simulink model "controller"  (R2022b)
settings: Solver=VariableStepAuto  StartTime=0.0  StopTime=10  RelTol=1e-3
values from neighbouring files (symbols this model uses):
  a_1 = x(25)    [disturbance_torque_generator.m]    (also in dynamic_terms.m = robot_parameters(9); dz_calculator.m; load_data.m = 0.5; nonlinear_disturbance_observer_controller.m)
  a_2 = x(26)    [disturbance_torque_generator.m]    (also in dynamic_terms.m = robot_parameters(10); dz_calculator.m; load_data.m = 0.4; nonlinear_disturbance_observer_controller.m)
  f_c1 = x(5)    [disturbance_torque_generator.m]    (also in load_data.m = 0.49)
  f_c2 = x(6)    [disturbance_torque_generator.m]    (also in load_data.m = 0.31)
  f_c3 = x(7)    [disturbance_torque_generator.m]    (also in load_data.m = 0.1)
  f_c4 = x(8)    [disturbance_torque_generator.m]    (also in load_data.m = 0.1)
  f_payload = x(27)    [disturbance_torque_generator.m]    (also in load_data.m = 2)
  f_s1 = x(9)    [disturbance_torque_generator.m]    (also in load_data.m = 3.5)
  f_s2 = x(10)    [disturbance_torque_generator.m]    (also in load_data.m = 2.8)
  f_s3 = x(11)    [disturbance_torque_generator.m]    (also in load_data.m = 1.65)
  f_s4 = x(12)    [disturbance_torque_generator.m]    (also in load_data.m = 0.7)
  f_v1 = x(13)    [disturbance_torque_generator.m]    (also in load_data.m = 0.15)
  f_v2 = x(14)    [disturbance_torque_generator.m]    (also in load_data.m = 0.12)
  f_v3 = x(15)    [disturbance_torque_generator.m]    (also in load_data.m = 0.08)
  f_v4 = x(16)    [disturbance_torque_generator.m]    (also in load_data.m = 0.03)
  I_1 = robot_parameters(5)    [dynamic_terms.m]    (also in dz_calculator.m = x(21); load_data.m = 0.31305; nonlinear_disturbance_observer_controller.m = x(21); open_loop_dynamics.m = x(17))
  I_2 = robot_parameters(6)    [dynamic_terms.m]    (also in dz_calculator.m = x(22); load_data.m = 0.96; nonlinear_disturbance_observer_controller.m = x(22); open_loop_dynamics.m = x(18))
  I_3 = robot_parameters(7)    [dynamic_terms.m]    (also in dz_calculator.m = x(23); load_data.m = 0.05; nonlinear_disturbance_observer_controller.m = x(23); open_loop_dynamics.m = x(19))
  I_4 = robot_parameters(8)    [dynamic_terms.m]    (also in dz_calculator.m = x(24); load_data.m = 0.06; nonlinear_disturbance_observer_controller.m = x(24); open_loop_dynamics.m = x(20))
  k_p = 2    [load_data.m]    (also in nonlinear_disturbance_observer_controller.m = x(30))
  k_v = 1.5    [load_data.m]    (also in nonlinear_disturbance_observer_controller.m = x(29))
  m_1 = robot_parameters(1)    [dynamic_terms.m]    (also in dz_calculator.m = x(17); load_data.m = 15; nonlinear_disturbance_observer_controller.m = x(17); open_loop_dynamics.m = x(13))
  m_2 = robot_parameters(2)    [dynamic_terms.m]    (also in dz_calculator.m = x(18); load_data.m = 12; nonlinear_disturbance_observer_controller.m = x(18); open_loop_dynamics.m = x(14))
  m_3 = robot_parameters(3)    [dynamic_terms.m]    (also in dz_calculator.m = x(19); load_data.m = 3; nonlinear_disturbance_observer_controller.m = x(19); open_loop_dynamics.m = x(15))
  m_4 = robot_parameters(4)    [dynamic_terms.m]    (also in dz_calculator.m = x(20); load_data.m = 3; nonlinear_disturbance_observer_controller.m = x(20); open_loop_dynamics.m = x(16))
  v_s1 = x(17)    [disturbance_torque_generator.m]    (also in load_data.m = 0.19)
  v_s2 = x(18)    [disturbance_torque_generator.m]    (also in load_data.m = 0.15)
  v_s3 = x(19)    [disturbance_torque_generator.m]    (also in load_data.m = 0.12)
  v_s4 = x(20)    [disturbance_torque_generator.m]    (also in load_data.m = 0.03)
  x_1 = robot_parameters(11)    [dynamic_terms.m]    (also in dz_calculator.m = x(27); load_data.m = 0.25; nonlinear_disturbance_observer_controller.m = x(27); open_loop_dynamics.m = x(23))
  x_2 = robot_parameters(12)    [dynamic_terms.m]    (also in dz_calculator.m = x(28); load_data.m = 0.2; nonlinear_disturbance_observer_controller.m = x(28); open_loop_dynamics.m = x(24))
  x_inv = x(5)    [dp_calculator.m]    (also in dz_calculator.m = x(29); load_data.m = 95.8)
libraries: simulink x8
settings Model: Creator=Mahdi  LastModifiedBy=Mahdi
settings SolverCC: MaxConsecutiveMinStep=10
settings DebuggingCC: UnderSpecifiedDimensionMsg=warning

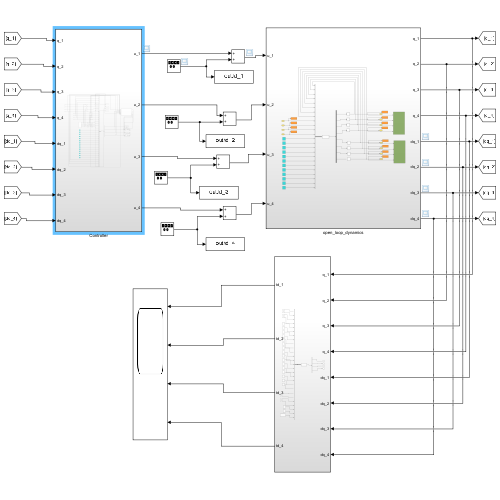
[thumbnail: Simulink's stored preview of the top-level diagram]
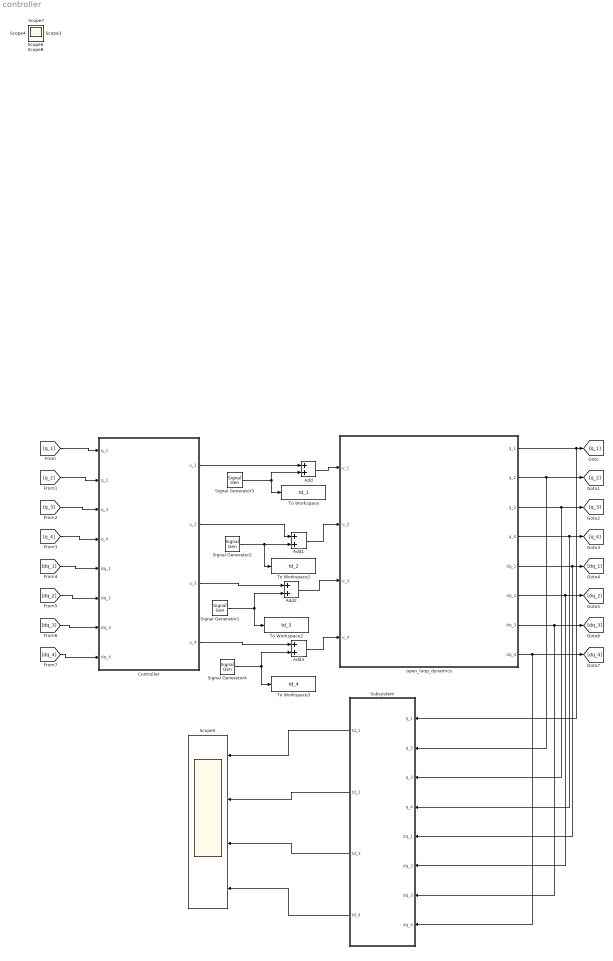
== system controller ==
  Add{,1..3} (4 alike) : Sum
  Controller : Subsystem
  Scope5 : Scope  NumInputPorts=4
  Signal Generator1 : SignalGenerator  Amplitude=0  Frequency=18  Units=rad/sec
  Signal Generator2 : SignalGenerator  Amplitude=-0.4  Frequency=0.8  Units=rad/sec
  Signal Generator3 : SignalGenerator  Amplitude=0.2  Frequency=0.27  Units=rad/sec
  Signal Generator4 : SignalGenerator  Amplitude=0  Frequency=4  Units=rad/sec
  Subsystem : Subsystem
  To Workspace : ToWorkspace  VariableName=td_1  SaveFormat=Timeseries  SampleTime=-1
  To Workspace1 : ToWorkspace  VariableName=td_2  SaveFormat=Timeseries  SampleTime=-1
  To Workspace2 : ToWorkspace  VariableName=td_3  SaveFormat=Timeseries  SampleTime=-1
  To Workspace3 : ToWorkspace  VariableName=td_4  SaveFormat=Timeseries  SampleTime=-1
  open_loop_dynamics : Subsystem
  Scope{,1..4,6..8} (8 alike) : Scope
  wires:
  [q_1] -> Controller/1(q_1)
  [q_2] -> Controller/2(q_2)
  [q_3] -> Controller/3(q_3)
  [q_4] -> Controller/4(q_4)
  [dq_1] -> Controller/5(dq_1)
  [dq_2] -> Controller/6(dq_2)
  [dq_3] -> Controller/7(dq_3)
  [dq_4] -> Controller/8(dq_4)
  open_loop_dynamics/1(q_1) -> Subsystem/1(q_1), [q_1]
  open_loop_dynamics/2(q_2) -> [q_2], Subsystem/2(q_2)
  open_loop_dynamics/3(q_3) -> [q_3], Subsystem/3(q_3)
  open_loop_dynamics/4(q_4) -> [q_4], Subsystem/4(q_4)
  open_loop_dynamics/5(dq_1) -> [dq_1], Subsystem/5(dq_1)
  open_loop_dynamics/6(dq_2) -> [dq_2], Subsystem/6(dq_2)
  open_loop_dynamics/7(dq_3) -> [dq_3], Subsystem/7(dq_3)
  open_loop_dynamics/8(dq_4) -> [dq_4], Subsystem/8(dq_4)
  Signal Generator3/1 -> Add/2, To Workspace/1
  Signal Generator2/1 -> Add1/2, To Workspace1/1
  Signal Generator1/1 -> Add2/2, To Workspace2/1
  Controller/1(u_1) -> Add/1
  Controller/2(u_2) -> Add1/1
  Add/1 -> open_loop_dynamics/1(u_1)
  Add1/1 -> open_loop_dynamics/2(u_2)
  Add2/1 -> open_loop_dynamics/3(u_3)
  Controller/3(u_3) -> Add2/1
  Signal Generator4/1 -> Add3/2, To Workspace3/1
  Controller/4(u_4) -> Add3/1
  Add3/1 -> open_loop_dynamics/4(u_4)
  Subsystem/1(td_1) -> Scope5/1
  Subsystem/2(td_2) -> Scope5/2
  Subsystem/3(td_3) -> Scope5/3
  Subsystem/4(td_4) -> Scope5/4

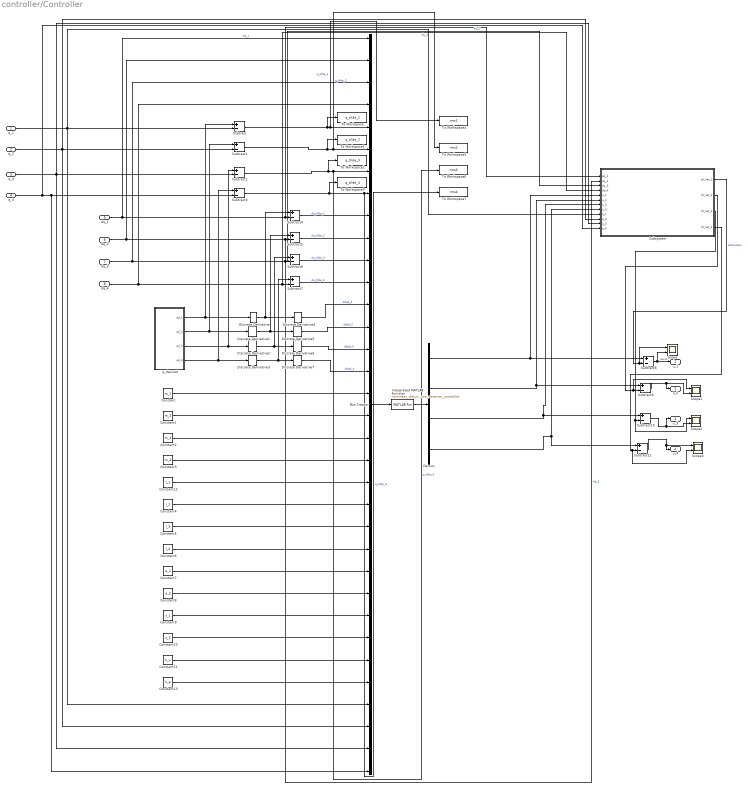
== system controller/Controller ==
  q_1 : Inport
  q_2 : Inport  Port=2
  q_3 : Inport  Port=3
  q_4 : Inport  Port=4
  dq_1 : Inport  Port=5
  dq_2 : Inport  Port=6
  dq_3 : Inport  Port=7
  dq_4 : Inport  Port=8
  Bus Creator : BusCreator  Inputs=34
  Constant : Constant  Value=m_1
  Constant1 : Constant  Value=m_2
  Constant10 : Constant  Value=x_2
  Constant11 : Constant  Value=k_v
  Constant12 : Constant  Value=I_1
  Constant13 : Constant  Value=k_p
  Constant2 : Constant  Value=m_3
  Constant3 : Constant  Value=m_4
  Constant4 : Constant  Value=I_2
  Constant5 : Constant  Value=I_3
  Constant6 : Constant  Value=I_4
  Constant7 : Constant  Value=a_1
  Constant8 : Constant  Value=a_2
  Constant9 : Constant  Value=x_1
  Demux : Demux
  Discrete Derivative{,1..7} (8 alike) : simulink/Discrete/Discrete Derivative  gainval=1.0  ICPrevScaledInput=0.0  OutMin=[]  OutMax=[]  OutDataType=fixdt(1, 16)  OutScaling=2^-10  DoSatur=off
  Interpreted MATLAB Function : MATLABFcn  MATLABFcn=nonlinear_disturbance_observer_controller
  Scope{,1..3} (4 alike) : Scope  NumInputPorts=2
  Subsystem : Subsystem
  Subtract{,1..11} (12 alike) : Sum  Inputs=+-
  To Workspace : ToWorkspace  VariableName=q_tilde_1  SaveFormat=Timeseries  SampleTime=-1
  To Workspace1 : ToWorkspace  VariableName=q_tilde_2  SaveFormat=Timeseries  SampleTime=-1
  To Workspace2 : ToWorkspace  VariableName=q_tilde_3  SaveFormat=Timeseries  SampleTime=-1
  To Workspace3 : ToWorkspace  VariableName=q_tilde_4  SaveFormat=Timeseries  SampleTime=-1
  To Workspace4 : ToWorkspace  VariableName=rms1  SampleTime=-1
      settings: Save2DSignal=2-D array (concatenate along first dimension)
  To Workspace5 : ToWorkspace  VariableName=rms2  SampleTime=-1
      settings: Save2DSignal=2-D array (concatenate along first dimension)
  To Workspace6 : ToWorkspace  VariableName=rms3  SampleTime=-1
      settings: Save2DSignal=2-D array (concatenate along first dimension)
  To Workspace7 : ToWorkspace  VariableName=rms4  SampleTime=-1
      settings: Save2DSignal=2-D array (concatenate along first dimension)
  q_desired : Subsystem
  u_1 : Outport
  u_2 : Outport  Port=2
  u_3 : Outport  Port=3
  u_4 : Outport  Port=4
  wires:
  dq_2/1 -> Bus Creator/2, Subsystem/2(dq_2), Subtract5/2  "dq_2"
  dq_1/1 -> Bus Creator/1, Subsystem/1(dq_1), Subtract4/2  "dq_1"
  q_desired/1(qd_1) -> Discrete Derivative/1, Subtract/1
  q_desired/4(qd_4) -> Discrete Derivative3/1, Subtract3/1
  dq_3/1 -> Bus Creator/3, Subsystem/3(dq_3), Subtract6/2  "dq_3"
  Discrete Derivative5/1 -> Bus Creator/14  "ddqd_2"
  Discrete Derivative/1 -> Discrete Derivative4/1, Subtract4/1
  Discrete Derivative3/1 -> Discrete Derivative7/1, Subtract7/1
  Subtract3/1 -> To Workspace7/1, Bus Creator/8, To Workspace3/1  "q_tilde_4"
  Interpreted MATLAB Function/1 -> Demux/1
  Constant3/1 -> Bus Creator/20
  q_desired/2(qd_2) -> Discrete Derivative1/1, Subtract1/1
  q_1/1 -> Subtract/2, Bus Creator/31, Subsystem/9(q_1)
  Constant/1 -> Bus Creator/17
  Constant12/1 -> Bus Creator/21
  Constant6/1 -> Bus Creator/24
  Constant2/1 -> Bus Creator/19
  Subtract4/1 -> Bus Creator/9  "dq_tilde_1"
  Constant9/1 -> Bus Creator/27
  Subtract6/1 -> Bus Creator/11  "dq_tilde_3"
  Discrete Derivative6/1 -> Bus Creator/15  "ddqd_3"
  Constant5/1 -> Bus Creator/23
  dq_4/1 -> Bus Creator/4, Subtract7/2, Subsystem/4(dq_4)  "dq_4"
  Constant11/1 -> Bus Creator/29
  Constant4/1 -> Bus Creator/22
  Discrete Derivative7/1 -> Bus Creator/16  "ddqd_4"
  Discrete Derivative4/1 -> Bus Creator/13  "ddqd_1"
  Constant8/1 -> Bus Creator/26
  Subtract5/1 -> Bus Creator/10  "dq_tilde_2"
  Discrete Derivative1/1 -> Discrete Derivative5/1, Subtract5/1
  q_3/1 -> Subtract2/2, Bus Creator/33, Subsystem/11(q_3)
  Subtract1/1 -> To Workspace1/1, Bus Creator/6, To Workspace5/1  "q_tilde_2"
  Subtract7/1 -> Bus Creator/12  "dq_tilde_4"
  Subtract/1 -> To Workspace4/1, Bus Creator/5, To Workspace/1  "q_tilde_1"
  q_4/1 -> Subsystem/12(q_4), Bus Creator/34, Subtract3/2
  q_desired/3(qd_3) -> Discrete Derivative2/1, Subtract2/1
  Discrete Derivative2/1 -> Discrete Derivative6/1, Subtract6/1
  Constant10/1 -> Bus Creator/28
  q_2/1 -> Subtract1/2, Bus Creator/32, Subsystem/10(q_2)
  Subtract2/1 -> To Workspace6/1, Bus Creator/7, To Workspace2/1  "q_tilde_3"
  Constant1/1 -> Bus Creator/18
  Constant7/1 -> Bus Creator/25
  Constant13/1 -> Bus Creator/30
  Bus Creator/1 -> Interpreted MATLAB Function/1
  Demux/1 -> Subtract8/1, Subsystem/5(u_1)
  Subsystem/1(td_hat_1) -> Scope/1, Subtract8/2  "estimation"
  Demux/2 -> Subtract9/1, Subsystem/6(u_2)
  Demux/3 -> Subtract10/1, Subsystem/7(u_3)
  Demux/4 -> Subtract11/1, Subsystem/8(u_4)
  Subsystem/2(td_hat_2) -> Subtract9/2, Scope1/1
  Subsystem/3(td_hat_3) -> Scope2/1, Subtract10/2
  Subsystem/4(td_hat_4) -> Scope3/2, Subtract11/2
  Subtract8/1 -> u_1/1, Scope/2  "result"
  Subtract10/1 -> u_3/1, Scope2/2
  Subtract9/1 -> u_2/1, Scope1/2
  Subtract11/1 -> u_4/1, Scope3/1

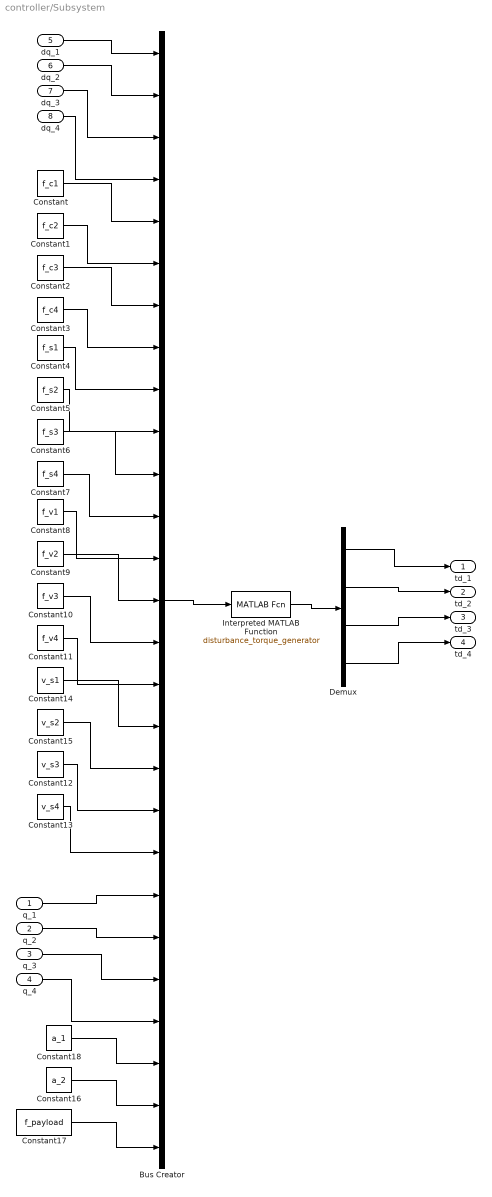
== system controller/Subsystem ==
  q_1 : Inport
  q_2 : Inport  Port=2
  q_3 : Inport  Port=3
  q_4 : Inport  Port=4
  dq_1 : Inport  Port=5
  dq_2 : Inport  Port=6
  dq_3 : Inport  Port=7
  dq_4 : Inport  Port=8
  Bus Creator : BusCreator  Inputs=27
  Constant : Constant  Value=f_c1
  Constant1 : Constant  Value=f_c2
  Constant10 : Constant  Value=f_v3
  Constant11 : Constant  Value=f_v4
  Constant12 : Constant  Value=v_s3
  Constant13 : Constant  Value=v_s4
  Constant14 : Constant  Value=v_s1
  Constant15 : Constant  Value=v_s2
  Constant16 : Constant  Value=a_2
  Constant17 : Constant  Value=f_payload
  Constant18 : Constant  Value=a_1
  Constant2 : Constant  Value=f_c3
  Constant3 : Constant  Value=f_c4
  Constant4 : Constant  Value=f_s1
  Constant5 : Constant  Value=f_s2
  Constant6 : Constant  Value=f_s3
  Constant7 : Constant  Value=f_s4
  Constant8 : Constant  Value=f_v1
  Constant9 : Constant  Value=f_v2
  Demux : Demux
  Interpreted MATLAB Function : MATLABFcn  MATLABFcn=disturbance_torque_generator
  td_1 : Outport
  td_2 : Outport  Port=2
  td_3 : Outport  Port=3
  td_4 : Outport  Port=4
  wires:
  Constant/1 -> Bus Creator/5
  Constant1/1 -> Bus Creator/6
  Constant2/1 -> Bus Creator/7
  Constant3/1 -> Bus Creator/8
  Constant4/1 -> Bus Creator/9
  Constant5/1 -> Bus Creator/10
  Constant6/1 -> Bus Creator/11
  Constant7/1 -> Bus Creator/12
  Constant8/1 -> Bus Creator/13
  Constant9/1 -> Bus Creator/14
  Constant10/1 -> Bus Creator/15
  Constant11/1 -> Bus Creator/16
  Constant14/1 -> Bus Creator/17
  Constant15/1 -> Bus Creator/18
  Constant12/1 -> Bus Creator/19
  Constant13/1 -> Bus Creator/20
  Constant17/1 -> Bus Creator/27
  Constant16/1 -> Bus Creator/26
  Constant18/1 -> Bus Creator/25
  dq_1/1 -> Bus Creator/1
  dq_2/1 -> Bus Creator/2
  dq_3/1 -> Bus Creator/3
  dq_4/1 -> Bus Creator/4
  q_1/1 -> Bus Creator/21
  q_2/1 -> Bus Creator/22
  q_3/1 -> Bus Creator/23
  q_4/1 -> Bus Creator/24
  Bus Creator/1 -> Interpreted MATLAB Function/1
  Interpreted MATLAB Function/1 -> Demux/1
  Demux/1 -> td_1/1
  Demux/2 -> td_2/1
  Demux/3 -> td_3/1
  Demux/4 -> td_4/1

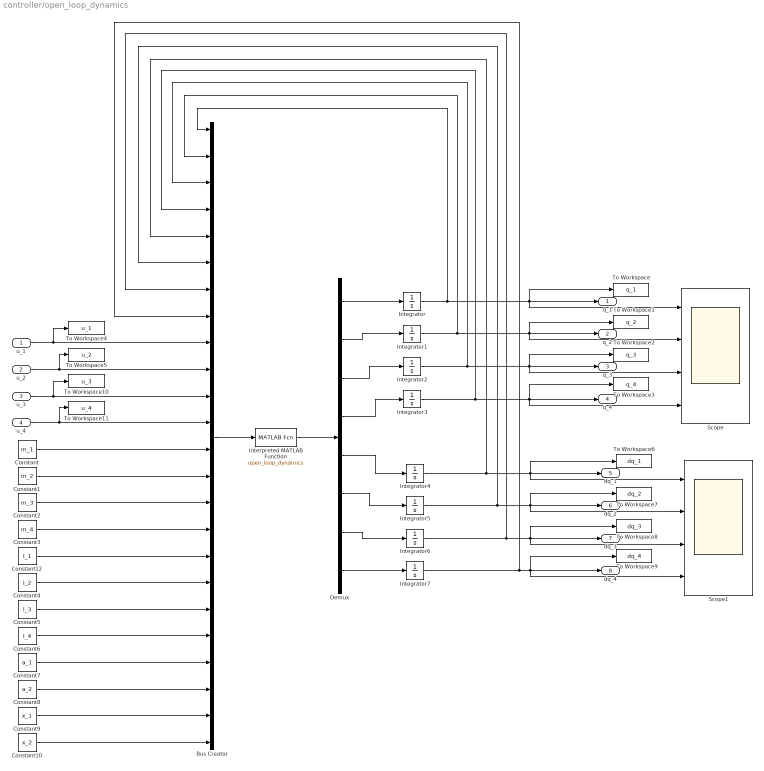
== system controller/open_loop_dynamics ==
  u_1 : Inport
  u_2 : Inport  Port=2
  u_3 : Inport  Port=3
  u_4 : Inport  Port=4
  Bus Creator : BusCreator  Inputs=24
  Constant : Constant  Value=m_1
  Constant1 : Constant  Value=m_2
  Constant10 : Constant  Value=x_2
  Constant12 : Constant  Value=I_1
  Constant2 : Constant  Value=m_3
  Constant3 : Constant  Value=m_4
  Constant4 : Constant  Value=I_2
  Constant5 : Constant  Value=I_3
  Constant6 : Constant  Value=I_4
  Constant7 : Constant  Value=a_1
  Constant8 : Constant  Value=a_2
  Constant9 : Constant  Value=x_1
  Demux : Demux  Outputs=8
  Integrator{,1..7} (8 alike) : Integrator
  Interpreted MATLAB Function : MATLABFcn  MATLABFcn=open_loop_dynamics
  Scope : Scope  NumInputPorts=4
  Scope1 : Scope  NumInputPorts=4
  To Workspace : ToWorkspace  VariableName=q_1  SampleTime=-1
  To Workspace1 : ToWorkspace  VariableName=q_2  SampleTime=-1
  To Workspace10 : ToWorkspace  VariableName=u_3  SampleTime=-1
  To Workspace11 : ToWorkspace  VariableName=u_4  SampleTime=-1
  To Workspace2 : ToWorkspace  VariableName=q_3  SampleTime=-1
  To Workspace3 : ToWorkspace  VariableName=q_4  SampleTime=-1
  To Workspace4 : ToWorkspace  VariableName=u_1  SampleTime=-1
  To Workspace5 : ToWorkspace  VariableName=u_2  SampleTime=-1
  To Workspace6 : ToWorkspace  VariableName=dq_1  SampleTime=-1
  To Workspace7 : ToWorkspace  VariableName=dq_2  SampleTime=-1
  To Workspace8 : ToWorkspace  VariableName=dq_3  SampleTime=-1
  To Workspace9 : ToWorkspace  VariableName=dq_4  SampleTime=-1
  q_1 : Outport
  q_2 : Outport  Port=2
  q_3 : Outport  Port=3
  q_4 : Outport  Port=4
  dq_1 : Outport  Port=5
  dq_2 : Outport  Port=6
  dq_3 : Outport  Port=7
  dq_4 : Outport  Port=8
  wires:
  Integrator6/1 -> dq_3/1, Scope1/3, To Workspace8/1, Bus Creator/7
  Integrator/1 -> q_1/1, To Workspace/1, Scope/1, Bus Creator/1
  Constant3/1 -> Bus Creator/16
  Integrator4/1 -> dq_1/1, Scope1/1, To Workspace6/1, Bus Creator/5
  Constant5/1 -> Bus Creator/19
  u_2/1 -> To Workspace5/1, Bus Creator/10
  Demux/3 -> Integrator2/1
  u_4/1 -> Bus Creator/12, To Workspace11/1
  Constant4/1 -> Bus Creator/18
  u_1/1 -> Bus Creator/9, To Workspace4/1
  Demux/4 -> Integrator3/1
  Integrator2/1 -> q_3/1, To Workspace2/1, Scope/3, Bus Creator/3
  Integrator3/1 -> q_4/1, To Workspace3/1, Scope/4, Bus Creator/4
  Integrator7/1 -> dq_4/1, Scope1/4, To Workspace9/1, Bus Creator/8
  Demux/1 -> Integrator/1
  Constant2/1 -> Bus Creator/15
  Demux/7 -> Integrator6/1
  Interpreted MATLAB Function/1 -> Demux/1
  Demux/2 -> Integrator1/1
  Integrator5/1 -> dq_2/1, Scope1/2, To Workspace7/1, Bus Creator/6
  Demux/8 -> Integrator7/1
  Demux/6 -> Integrator5/1
  Integrator1/1 -> q_2/1, To Workspace1/1, Scope/2, Bus Creator/2
  u_3/1 -> Bus Creator/11, To Workspace10/1
  Bus Creator/1 -> Interpreted MATLAB Function/1
  Demux/5 -> Integrator4/1
  Constant12/1 -> Bus Creator/17
  Constant6/1 -> Bus Creator/20
  Constant1/1 -> Bus Creator/14
  Constant/1 -> Bus Creator/13
  Constant7/1 -> Bus Creator/21
  Constant8/1 -> Bus Creator/22
  Constant9/1 -> Bus Creator/23
  Constant10/1 -> Bus Creator/24

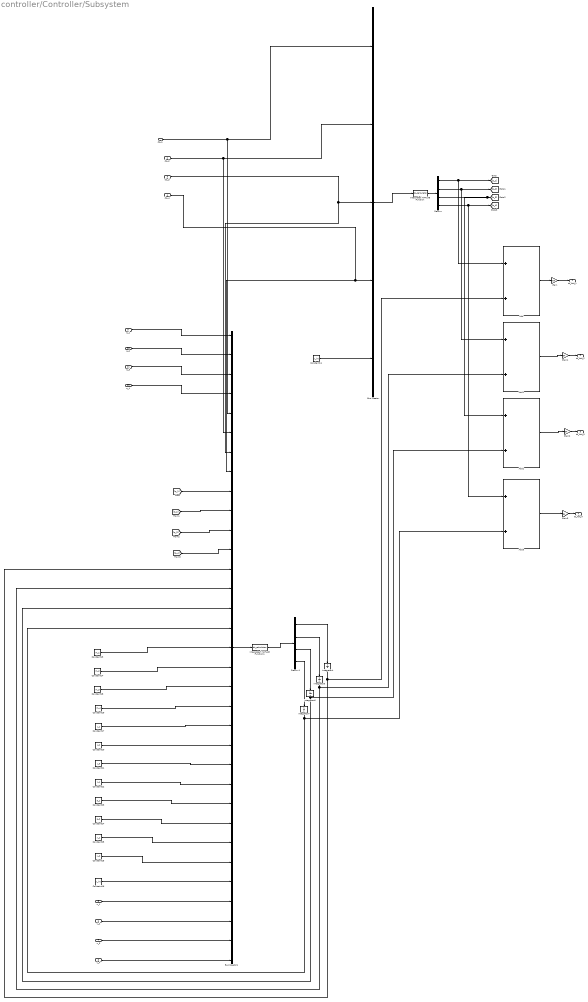
== system controller/Controller/Subsystem ==
  dq_1 : Inport
  dq_2 : Inport  Port=2
  dq_3 : Inport  Port=3
  dq_4 : Inport  Port=4
  u_1 : Inport  Port=5
  u_2 : Inport  Port=6
  u_3 : Inport  Port=7
  u_4 : Inport  Port=8
  q_1 : Inport  Port=9
  q_2 : Inport  Port=10
  q_3 : Inport  Port=11
  q_4 : Inport  Port=12
  Add{,1..3} (4 alike) : Sum
  Bus Creator : BusCreator  Inputs=5
  Bus Creator1 : BusCreator  Inputs=33
  Constant11 : Constant  Value=x_inv
  Constant13 : Constant  Value=m_1
  Constant14 : Constant  Value=m_2
  Constant15 : Constant  Value=x_2
  Constant16 : Constant  Value=x_inv
  Constant17 : Constant  Value=I_1
  Constant18 : Constant  Value=m_3
  Constant19 : Constant  Value=m_4
  Constant20 : Constant  Value=I_2
  Constant21 : Constant  Value=I_3
  Constant22 : Constant  Value=I_4
  Constant23 : Constant  Value=a_1
  Constant24 : Constant  Value=a_2
  Constant25 : Constant  Value=x_1
  Demux : Demux
  Demux1 : Demux
  Gain{,1..3} (4 alike) : Gain  Gain=64
  Integrator{4..7} (4 alike) : Integrator
  Interpreted MATLAB Function : MATLABFcn  MATLABFcn=dp_calculator
  Interpreted MATLAB Function1 : MATLABFcn  MATLABFcn=dz_calculator
  td_hat_1 : Outport
  td_hat_2 : Outport  Port=2
  td_hat_3 : Outport  Port=3
  td_hat_4 : Outport  Port=4
  wires:
  Interpreted MATLAB Function/1 -> Demux/1
  dq_2/1 -> Bus Creator/2, Bus Creator1/6
  dq_3/1 -> Bus Creator1/7, Bus Creator/3
  Bus Creator/1 -> Interpreted MATLAB Function/1
  dq_1/1 -> Bus Creator1/5, Bus Creator/1
  Bus Creator1/1 -> Interpreted MATLAB Function1/1
  Interpreted MATLAB Function1/1 -> Demux1/1
  Demux1/1 -> Integrator4/1
  Demux1/2 -> Integrator5/1
  Demux1/3 -> Integrator6/1
  Demux1/4 -> Integrator7/1
  Constant13/1 -> Bus Creator1/17
  Constant14/1 -> Bus Creator1/18
  Constant18/1 -> Bus Creator1/19
  Constant19/1 -> Bus Creator1/20
  Constant17/1 -> Bus Creator1/21
  Constant20/1 -> Bus Creator1/22
  Constant21/1 -> Bus Creator1/23
  Constant22/1 -> Bus Creator1/24
  Constant23/1 -> Bus Creator1/25
  Constant24/1 -> Bus Creator1/26
  Constant25/1 -> Bus Creator1/27
  Constant15/1 -> Bus Creator1/28
  Constant16/1 -> Bus Creator1/29
  u_1/1 -> Bus Creator1/30
  u_2/1 -> Bus Creator1/31
  u_3/1 -> Bus Creator1/32
  u_4/1 -> Bus Creator1/33
  Integrator4/1 -> Add/2, Bus Creator1/13
  Integrator5/1 -> Bus Creator1/14, Add1/2
  Integrator6/1 -> Add2/2, Bus Creator1/15
  Integrator7/1 -> Add3/2, Bus Creator1/16
  [p_4] -> Bus Creator1/12
  [p_3] -> Bus Creator1/11
  [p_2] -> Bus Creator1/10
  [p_1] -> Bus Creator1/9
  Demux/1 -> [p_1], Add/1
  Demux/2 -> [p_2], Add1/1
  Demux/4 -> [p_4], Add3/1
  Demux/3 -> Add2/1, [p_3]
  dq_4/1 -> Bus Creator1/8, Bus Creator/4
  Constant11/1 -> Bus Creator/5
  q_1/1 -> Bus Creator1/1
  q_2/1 -> Bus Creator1/2
  q_3/1 -> Bus Creator1/3
  q_4/1 -> Bus Creator1/4
  Add/1 -> Gain/1
  Add1/1 -> Gain1/1
  Add2/1 -> Gain2/1
  Add3/1 -> Gain3/1
  Gain/1 -> td_hat_1/1
  Gain1/1 -> td_hat_2/1
  Gain2/1 -> td_hat_3/1
  Gain3/1 -> td_hat_4/1

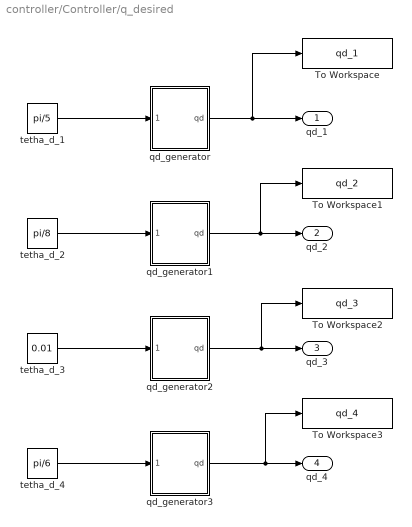
== system controller/Controller/q_desired ==
  To Workspace : ToWorkspace  VariableName=qd_1  SaveFormat=Timeseries  SampleTime=-1
  To Workspace1 : ToWorkspace  VariableName=qd_2  SaveFormat=Timeseries  SampleTime=-1
  To Workspace2 : ToWorkspace  VariableName=qd_3  SaveFormat=Timeseries  SampleTime=-1
  To Workspace3 : ToWorkspace  VariableName=qd_4  SaveFormat=Timeseries  SampleTime=-1
  qd_generator : Subsystem
  qd_generator1 : Subsystem
  qd_generator2 : Subsystem
  qd_generator3 : Subsystem
  tetha_d_1 : Constant  Value=pi/5
  tetha_d_2 : Constant  Value=pi/8
  tetha_d_3 : Constant  Value=0.01
  tetha_d_4 : Constant  Value=pi/6
  qd_1 : Outport
  qd_2 : Outport  Port=2
  qd_3 : Outport  Port=3
  qd_4 : Outport  Port=4
  wires:
  tetha_d_3/1 -> qd_generator2/1(tetha_d)
  qd_generator2/1(qd) -> qd_3/1, To Workspace2/1
  qd_generator/1(qd) -> To Workspace/1, qd_1/1
  qd_generator3/1(qd) -> qd_4/1, To Workspace3/1
  qd_generator1/1(qd) -> qd_2/1, To Workspace1/1
  tetha_d_1/1 -> qd_generator/1(tetha_d)
  tetha_d_4/1 -> qd_generator3/1(tetha_d)
  tetha_d_2/1 -> qd_generator1/1(tetha_d)

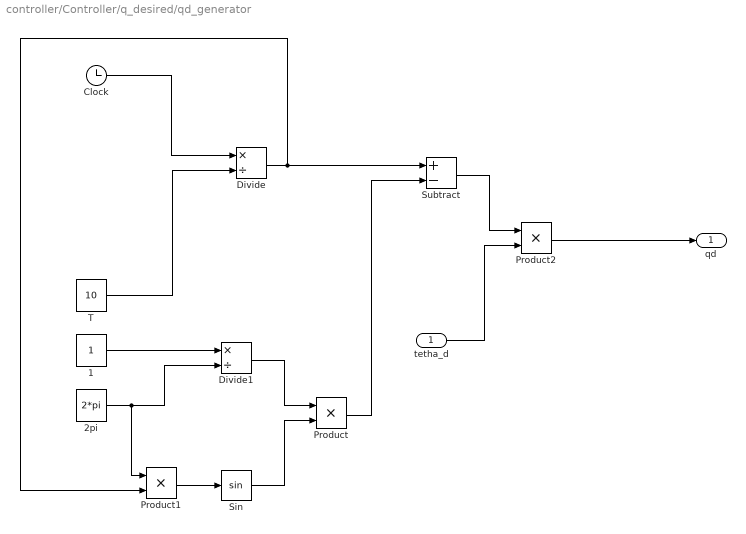
== system controller/Controller/q_desired/qd_generator ==
  tetha_d : Inport
  1 : Constant
  2pi : Constant  Value=2*pi
  Clock : Clock
  Divide : Product  Inputs=*/
  Divide1 : Product  Inputs=*/
  Product : Product
  Product1 : Product
  Product2 : Product
  Sin : Trigonometry
  Subtract : Sum  Inputs=+-
  T : Constant  Value=10
  qd : Outport
  wires:
  Clock/1 -> Divide/1
  Product2/1 -> qd/1
  Divide1/1 -> Product/1
  Sin/1 -> Product/2
  T/1 -> Divide/2
  Product/1 -> Subtract/2
  tetha_d/1 -> Product2/2
  2pi/1 -> Product1/1, Divide1/2
  1/1 -> Divide1/1
  Divide/1 -> Product1/2, Subtract/1
  Product1/1 -> Sin/1
  Subtract/1 -> Product2/1

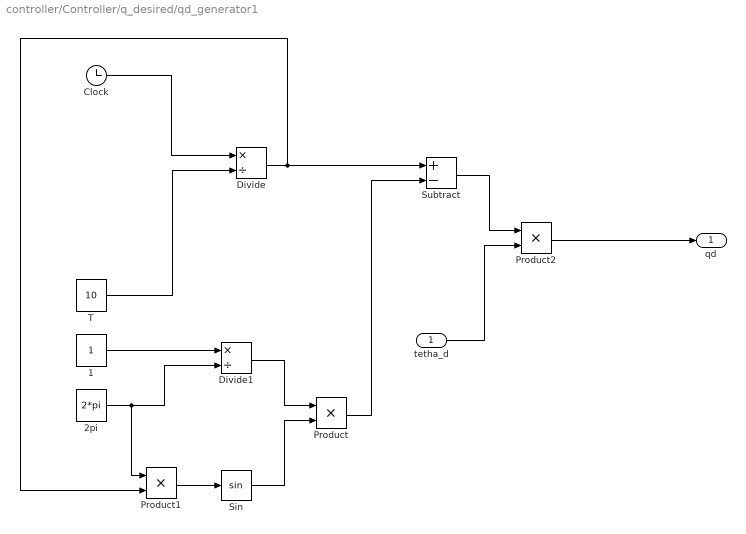
== system controller/Controller/q_desired/qd_generator1 ==
  tetha_d : Inport
  1 : Constant
  2pi : Constant  Value=2*pi
  Clock : Clock
  Divide : Product  Inputs=*/
  Divide1 : Product  Inputs=*/
  Product : Product
  Product1 : Product
  Product2 : Product
  Sin : Trigonometry
  Subtract : Sum  Inputs=+-
  T : Constant  Value=10
  qd : Outport
  wires:
  Subtract/1 -> Product2/1
  Product1/1 -> Sin/1
  Divide/1 -> Subtract/1, Product1/2
  1/1 -> Divide1/1
  2pi/1 -> Divide1/2, Product1/1
  tetha_d/1 -> Product2/2
  Product/1 -> Subtract/2
  T/1 -> Divide/2
  Sin/1 -> Product/2
  Divide1/1 -> Product/1
  Product2/1 -> qd/1
  Clock/1 -> Divide/1

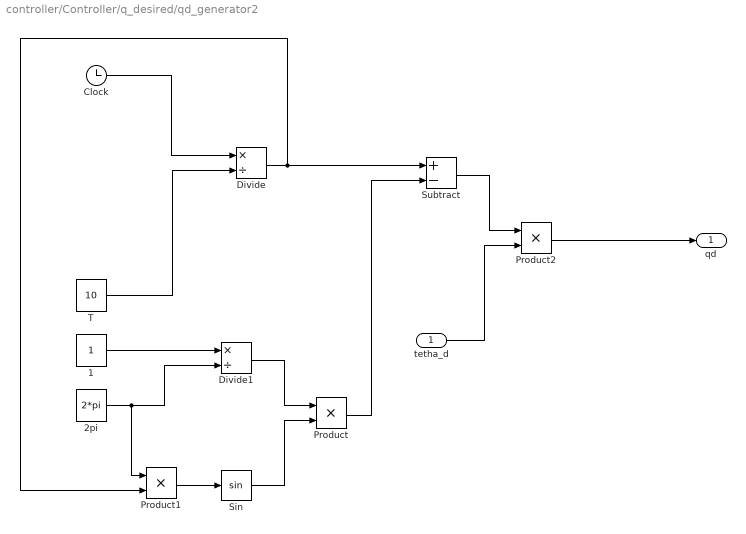
== system controller/Controller/q_desired/qd_generator2 ==
  tetha_d : Inport
  1 : Constant
  2pi : Constant  Value=2*pi
  Clock : Clock
  Divide : Product  Inputs=*/
  Divide1 : Product  Inputs=*/
  Product : Product
  Product1 : Product
  Product2 : Product
  Sin : Trigonometry
  Subtract : Sum  Inputs=+-
  T : Constant  Value=10
  qd : Outport
  wires:
  Clock/1 -> Divide/1
  Product2/1 -> qd/1
  Divide1/1 -> Product/1
  Sin/1 -> Product/2
  T/1 -> Divide/2
  Product/1 -> Subtract/2
  tetha_d/1 -> Product2/2
  2pi/1 -> Product1/1, Divide1/2
  1/1 -> Divide1/1
  Divide/1 -> Product1/2, Subtract/1
  Product1/1 -> Sin/1
  Subtract/1 -> Product2/1

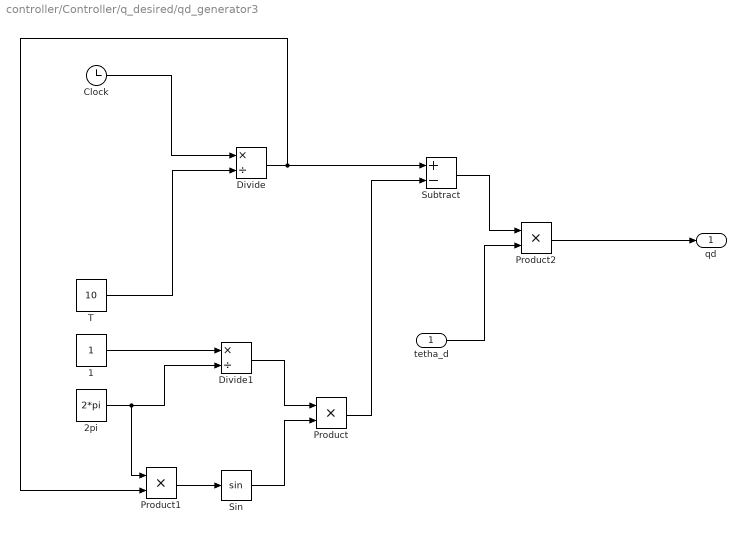
== system controller/Controller/q_desired/qd_generator3 ==
  tetha_d : Inport
  1 : Constant
  2pi : Constant  Value=2*pi
  Clock : Clock
  Divide : Product  Inputs=*/
  Divide1 : Product  Inputs=*/
  Product : Product
  Product1 : Product
  Product2 : Product
  Sin : Trigonometry
  Subtract : Sum  Inputs=+-
  T : Constant  Value=10
  qd : Outport
  wires:
  Subtract/1 -> Product2/1
  Product1/1 -> Sin/1
  Divide/1 -> Subtract/1, Product1/2
  1/1 -> Divide1/1
  2pi/1 -> Divide1/2, Product1/1
  tetha_d/1 -> Product2/2
  Product/1 -> Subtract/2
  T/1 -> Divide/2
  Sin/1 -> Product/2
  Divide1/1 -> Product/1
  Product2/1 -> qd/1
  Clock/1 -> Divide/1
